simulink model "SistemaGrua021"  (R2020b)
settings: Solver=VariableStepAuto  StartTime=0.0  StopTime=10  RelTol=1e-3
values from neighbouring files (symbols this model uses):
  bcx = 1e6    (= 1000000)    [Valores_1.m]    (also in valoresPlanta.m; valoresPlanta_29_9_24.m; valoresPlanta_V3.m; valoresPlanta_v4.m)
  bcy = 1e7    (= 10000000)    [Valores_1.m]    (also in valoresPlanta.m; valoresPlanta_29_9_24.m; valoresPlanta_V3.m; valoresPlanta_v4.m)
  beq = bt+(btd+btm*it^2)/rtd^2    (= 21697.2)    [Valores.m]    (also in Valores_1.m; valoresPlanta_29_9_24.m; valoresPlanta_v4.m)
  bh_eq = bhm*ih^2+bhd    (= 8720)    [Valores.m]    (also in Valores_1.m; valoresPlanta.m; valoresPlanta_29_9_24.m; valoresPlanta_V3.m)
  bhb = 1e8    (= 100000000)    [Valores.m]    (also in Valores_1.m; valoresPlanta.m; valoresPlanta_29_9_24.m; valoresPlanta_V3.m)
  bhEb = 2.2e9    (= 2200000000)    [Valores.m]    (also in Valores_1.m; valoresPlanta.m; valoresPlanta_29_9_24.m; valoresPlanta_V3.m)
  btb = 5e6    (= 5000000)    [Valores.m]    (also in Valores_1.m; valoresPlanta.m; valoresPlanta_29_9_24.m; valoresPlanta_V3.m)
  bwu = 150    [Valores.m]    (also in Valores_1.m; valoresPlanta.m; valoresPlanta_29_9_24.m; valoresPlanta_V3.m)
  g = 9.80665    [Valores.m]    (also in Valores_1.m; valoresPlanta.m; valoresPlanta_29_9_24.m; valoresPlanta_V3.m)
  ih = 22    [Valores.m]    (also in Valores_1.m; valoresPlanta.m; valoresPlanta_29_9_24.m; valoresPlanta_V3.m)
  it = 30    [Valores.m]    (also in Valores_1.m; valoresPlanta.m; valoresPlanta_29_9_24.m; valoresPlanta_V3.m)
  Jh_eq = Jhm_hb*ih^2+Jhd_hEb    (= 18320)    [Valores.m]    (also in Valores_1.m; valoresPlanta.m; valoresPlanta_29_9_24.m; valoresPlanta_V3.m)
  kcy = 1.8e9    (= 1800000000)    [Valores_1.m]    (also in valoresPlanta.m; valoresPlanta_29_9_24.m; valoresPlanta_V3.m; valoresPlanta_v4.m)
  kwu = 2.36e8    (= 236000000)    [Valores.m]    (also in Valores_1.m; valoresPlanta.m; valoresPlanta_29_9_24.m; valoresPlanta_V3.m)
  Mc_max = 5e4    (= 50000)    [Valores.m]    (also in Valores_1.m; valoresPlanta.m; valoresPlanta_29_9_24.m; valoresPlanta_V3.m)
  Mc_min = 2e3    (= 2000)    [Valores.m]    (also in Valores_1.m; valoresPlanta.m; valoresPlanta_29_9_24.m; valoresPlanta_V3.m)
  Meq = Mt+(it^2*Jtm_tb+Jtd)/rtd^2    (= 60000)    [Valores.m]    (also in Valores_1.m; valoresPlanta_29_9_24.m; valoresPlanta_v4.m)
  rhd = 0.75    [Valores.m]    (also in Valores_1.m; valoresPlanta.m; valoresPlanta_29_9_24.m; valoresPlanta_V3.m)
  rtd = 0.5    [Valores.m]    (also in Valores_1.m; valoresPlanta.m; valoresPlanta_29_9_24.m; valoresPlanta_V3.m)
  tau_tm = 1e-3    (= 0.001)    [Valores.m]    (also in Valores_1.m; valoresPlanta.m; valoresPlanta_29_9_24.m; valoresPlanta_V3.m)
  tauhm = 1e-3    (= 0.001)    [Valores.m]    (also in Valores_1.m)
  Thb_Max = 5e4    (= 50000)    [Valores.m]    (also in Valores_1.m; valoresPlanta.m; valoresPlanta_29_9_24.m; valoresPlanta_V3.m)
  ThEb_Max = 1.1e6    (= 1100000)    [Valores.m]    (also in Valores_1.m; valoresPlanta.m; valoresPlanta_29_9_24.m; valoresPlanta_V3.m)
  Thm_Max = 2e4    (= 20000)    [Valores.m]    (also in Valores_1.m; valoresPlanta.m; valoresPlanta_29_9_24.m; valoresPlanta_V3.m)
  Ttb_Max = 5e3    (= 5000)    [Valores.m]    (also in Valores_1.m; valoresPlanta.m; valoresPlanta_29_9_24.m; valoresPlanta_V3.m)
  Ttm_Max = 3e3    (= 3000)    [Valores.m]    (also in Valores_1.m; valoresPlanta.m; valoresPlanta_29_9_24.m = 4000; valoresPlanta_V3.m)
  Yt0 = 45    [Valores.m]    (also in Valores_1.m; valoresPlanta.m; valoresPlanta_29_9_24.m; valoresPlanta_V3.m)
undefined symbols (not defined in the file or in its folder): sigbuilder_block
settings Model: Creator=Matias  LastModifiedBy=Matias

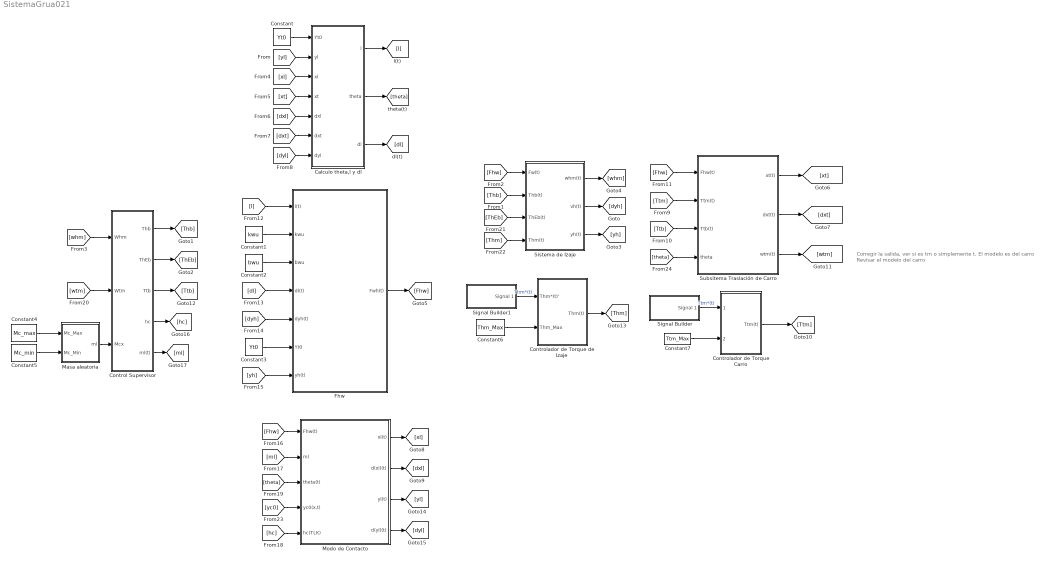
== system SistemaGrua021 ==
  note: Corregir la salida, ver si es tm o simplemente t. El modelo es del carro
      | Revisar el modelo del carro
  Calculo theta,l y dl : Subsystem
  Constant : Constant  Value=Yt0
  Constant1 : Constant  Value=kwu
  Constant2 : Constant  Value=bwu
  Constant3 : Constant  Value=Yt0
  Constant4 : Constant  Value=Mc_max
  Constant5 : Constant  Value=Mc_min
  Constant6 : Constant  Value=Thm_Max
  Constant7 : Constant  Value=Ttm_Max
  Control Supervisor : Subsystem
  Controlador de Torque Carro : Subsystem
  Controlador de Torque de Izaje : Subsystem
  Fhw : Subsystem
  Masa aleatoria : MATLAB Function  TreatAsAtomicUnit=on
  Modo de Contacto : Subsystem
  Signal Builder : Subsystem  Tag=STV Subsys  LoadFcn=sigbuilder_block('load');  StartFcn=sigbuilder_block('start');  StopFcn=sigbuilder_block('stop');  ClipboardFcn=sigbuilder_block('clipboard');  mask(Sigbuilder block){tuvar=[0:10]}
      mask help: Simulink:masks:SigbuilderBlock_MD
      mask init:
      | if ~strcmp(get_param(bdroot(gcbh),'SimulationStatus'),'stopped') tuvar = sigbuilder_block('maskInit'); end
      settings: CopyFcn=sigbuilder_block('copy');  DeleteFcn=sigbuilder_block('delete');  ModelCloseFcn=sigbuilder_block('modelClose');  PreSaveFcn=sigbuilder_block('preSave');  PauseFcn=sigbuilder_block('pause');  ContinueFcn=sigbuilder_block('continue');  NameChangeFcn=sigbuilder_block('namechange');  OpenFcn=sigbuilder_block('open',[5.4 36 1141.2 516.6 ]);  CloseFcn=sigbuilder_block('close');
      mask Display: plot(0, 0, 100, 100,[2, 2, 32, 32, 2], [68, 8, 8, 68, 68],[32, 2], [38, 38], [32, 19, 2],[53, 60, 44], [32, 17, 17, 2],[16, 16, 31, 31]);txt = getActiveGroup(gcbh);text(2, 100, txt,'verticalAlignment', 'top');
  Signal Builder1 : Subsystem  Tag=STV Subsys  LoadFcn=sigbuilder_block('load');  StartFcn=sigbuilder_block('start');  StopFcn=sigbuilder_block('stop');  ClipboardFcn=sigbuilder_block('clipboard');  mask(Sigbuilder block){tuvar=[0:10]}
      mask help: Simulink:masks:SigbuilderBlock_MD
      mask init:
      | if ~strcmp(get_param(bdroot(gcbh),'SimulationStatus'),'stopped') tuvar = sigbuilder_block('maskInit'); end
      settings: CopyFcn=sigbuilder_block('copy');  DeleteFcn=sigbuilder_block('delete');  ModelCloseFcn=sigbuilder_block('modelClose');  PreSaveFcn=sigbuilder_block('preSave');  PauseFcn=sigbuilder_block('pause');  ContinueFcn=sigbuilder_block('continue');  NameChangeFcn=sigbuilder_block('namechange');  OpenFcn=sigbuilder_block('open',[5.4 36 1141.2 516.6 ]);  CloseFcn=sigbuilder_block('close');
      mask Display: plot(0, 0, 100, 100,[2, 2, 32, 32, 2], [68, 8, 8, 68, 68],[32, 2], [38, 38], [32, 19, 2],[53, 60, 44], [32, 17, 17, 2],[16, 16, 31, 31]);txt = getActiveGroup(gcbh);text(2, 100, txt,'verticalAlignment', 'top');
  Sistema de Izaje : Subsystem
  Subsitema Traslación de Carro : Subsystem
  wires:
  [whm] -> Control Supervisor/1(Whm)
  Control Supervisor/1(Thb) -> [Thb]
  [Thb] -> Sistema de Izaje/2(Thb(t))
  [Fhw] -> Sistema de Izaje/1(Fw(t))
  Control Supervisor/2(ThEb) -> [ThEb]
  Calculo theta,l y dl/1(l) -> [l]
  Calculo theta,l y dl/2(theta) -> [theta]
  Constant/1 -> Calculo theta,l y dl/1(Yt0)
  [xt] -> Calculo theta,l y dl/4(xt)
  [xl] -> Calculo theta,l y dl/3(xl)
  [yl] -> Calculo theta,l y dl/2(yl)
  Calculo theta,l y dl/3(dl) -> [dl]
  [dyl] -> Calculo theta,l y dl/7(dyl)
  [dxt] -> Calculo theta,l y dl/6(dxt)
  [dxl] -> Calculo theta,l y dl/5(dxl)
  Fhw/1(Fwh(t)) -> [Fhw]
  [yh] -> Fhw/7(yh(t))
  [dyh] -> Fhw/5(dyh(t))
  [dl] -> Fhw/4(dl(t))
  [l] -> Fhw/1(l(t))
  Constant1/1 -> Fhw/2(kwu)
  Constant2/1 -> Fhw/3(bwu)
  [Ttb] -> Subsitema Traslación de Carro/3(Ttb(t))
  [Fhw] -> Subsitema Traslación de Carro/1(Fhw(t))
  [Ttm] -> Subsitema Traslación de Carro/2(Ttm(t))
  Subsitema Traslación de Carro/1(xt(t)) -> [xt]
  Subsitema Traslación de Carro/2(dxt(t)) -> [dxt]
  Controlador de Torque Carro/1(Ttm(t)) -> [Ttm]
  Signal Builder/1(Signal 1) -> Controlador de Torque Carro/1(Ttm*(t))  "Ttm*(t)"
  Subsitema Traslación de Carro/3(wtm(t)) -> [wtm]
  Control Supervisor/3(Ttb) -> [Ttb]
  [wtm] -> Control Supervisor/2(Wtm)
  Controlador de Torque de Izaje/1(Thm(t)) -> [Thm]
  Signal Builder1/1(Signal 1) -> Controlador de Torque de Izaje/1(Thm*(t)')  "Thm*(t)"
  Sistema de Izaje/1(whm(t)) -> [whm]
  Sistema de Izaje/2(vh(t)) -> [dyh]
  Sistema de Izaje/3(yh(t)) -> [yh]
  [ThEb] -> Sistema de Izaje/3(ThEb(t))
  [Thm] -> Sistema de Izaje/4(Thm(t))
  Constant3/1 -> Fhw/6(Yt0)
  Constant5/1 -> Masa aleatoria/2(Mc_Min)
  Constant4/1 -> Masa aleatoria/1(Mc_Max)
  Masa aleatoria/1(ml) -> Control Supervisor/3(Mcx)
  Constant6/1 -> Controlador de Torque de Izaje/2(Thm_Max)
  Constant7/1 -> Controlador de Torque Carro/2(Ttm_Max)
  [theta] -> Subsitema Traslación de Carro/4(theta)
  [yc0] -> Modo de Contacto/4(yc0(x,t))
  Modo de Contacto/2(d(xl)(t)) -> [dxl]
  Modo de Contacto/1(xl(t)) -> [xl]
  [hc] -> Modo de Contacto/5(hc(TLK))
  Modo de Contacto/4(d(yl)(t)) -> [dyl]
  [theta] -> Modo de Contacto/3(theta(t))
  Modo de Contacto/3(yl(t)) -> [yl]
  [ml] -> Modo de Contacto/2(ml)
  [Fhw] -> Modo de Contacto/1(Fhw(t))
  Control Supervisor/5(ml(t)) -> [ml]
  Control Supervisor/4(hc) -> [hc]

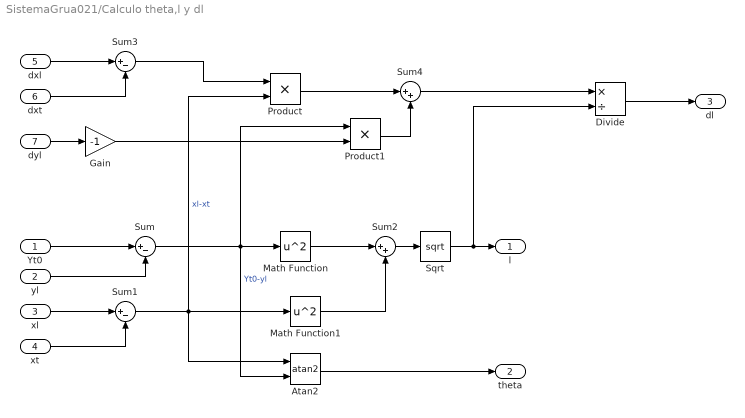
== system SistemaGrua021/Calculo theta,l y dl ==
  Yt0 : Inport
  yl : Inport  Port=2
  xl : Inport  Port=3
  xt : Inport  Port=4
  dxl : Inport  Port=5
  dxt : Inport  Port=6
  dyl : Inport  Port=7
  Atan2 : Trigonometry  Operator=atan2
  Divide : Product  Inputs=*/
  Gain : Gain  Gain=-1
  Math Function : Math  Operator=square  SaturateOnIntegerOverflow=on
  Math Function1 : Math  Operator=square  SaturateOnIntegerOverflow=on
  Product : Product
  Product1 : Product
  Sqrt : Sqrt  SaturateOnIntegerOverflow=on
  Sum : Sum  Inputs=|+-
  Sum1 : Sum  Inputs=|+-
  Sum2 : Sum  Inputs=|++
  Sum3 : Sum  Inputs=|+-
  Sum4 : Sum  Inputs=|++
  l : Outport
  theta : Outport  Port=2
  dl : Outport  Port=3
  wires:
  Yt0/1 -> Sum/1
  yl/1 -> Sum/2
  xl/1 -> Sum1/1
  xt/1 -> Sum1/2
  Atan2/1 -> theta/1
  Sum1/1 -> Product/2, Math Function1/1, Atan2/1  "xl-xt"
  Sum/1 -> Product1/1, Atan2/2, Math Function/1  "Yt0-yl"
  Math Function/1 -> Sum2/1
  Math Function1/1 -> Sum2/2
  Sum2/1 -> Sqrt/1
  Sqrt/1 -> Divide/2, l/1
  dxl/1 -> Sum3/1
  dxt/1 -> Sum3/2
  Sum3/1 -> Product/1
  dyl/1 -> Gain/1
  Gain/1 -> Product1/2
  Product/1 -> Sum4/1
  Product1/1 -> Sum4/2
  Sum4/1 -> Divide/1
  Divide/1 -> dl/1

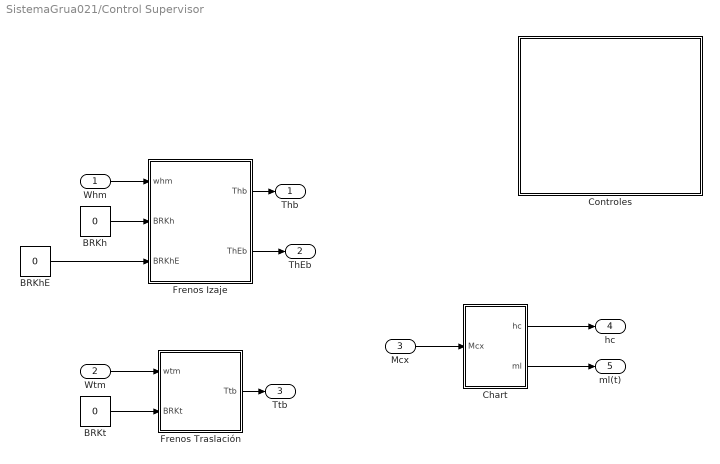
== system SistemaGrua021/Control Supervisor ==
  Whm : Inport
  Wtm : Inport  Port=2
  Mcx : Inport  Port=3
  BRKh : Constant  Value=0
  BRKhE : Constant  Value=0
  BRKt : Constant  Value=0
  Chart : Stateflow chart  TreatAsAtomicUnit=on
  Controles : Subsystem
  "Frenos Izaje " : Stateflow chart  TreatAsAtomicUnit=on
  Frenos Traslación : Stateflow chart  TreatAsAtomicUnit=on
  Thb : Outport
  ThEb : Outport  Port=2
  Ttb : Outport  Port=3
  hc : Outport  Port=4
  ml(t) : Outport  Port=5
  wires:
  "Frenos Izaje "/1(Thb) -> Thb/1
  BRKh/1 -> "Frenos Izaje "/2(BRKh)
  Whm/1 -> "Frenos Izaje "/1(whm)
  BRKhE/1 -> "Frenos Izaje "/3(BRKhE)
  "Frenos Izaje "/2(ThEb) -> ThEb/1
  Wtm/1 -> Frenos Traslación/1(wtm)
  Frenos Traslación/1(Ttb) -> Ttb/1
  BRKt/1 -> Frenos Traslación/2(BRKt)
  Chart/2(ml) -> ml(t)/1
  Chart/1(hc) -> hc/1
  Mcx/1 -> Chart/1(Mcx)

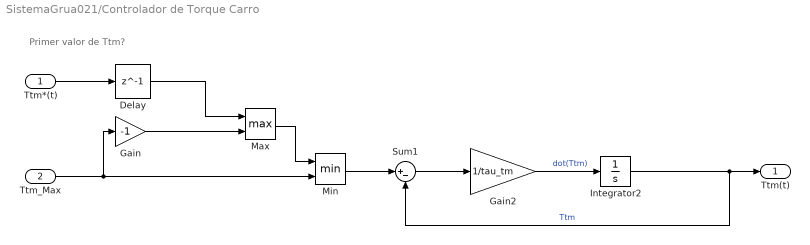
== system SistemaGrua021/Controlador de Torque Carro ==
  note: Primer valor de Ttm?
  Ttm*(t) : Inport
  Ttm_Max : Inport  Port=2
  Delay : Delay  DelayLength=1  InitialCondition=0
  Gain : Gain  Gain=-1
  Gain2 : Gain  Gain=1/tau_tm
  Integrator2 : Integrator
  Max : MinMax  Function=max  Inputs=2
  Min : MinMax  Inputs=2
  Sum1 : Sum  Inputs=|+-
  Ttm(t) : Outport
  wires:
  Integrator2/1 -> Ttm(t)/1, Sum1/2  "Ttm"
  Sum1/1 -> Gain2/1
  Gain2/1 -> Integrator2/1  "dot(Ttm)"
  Ttm*(t)/1 -> Delay/1
  Gain/1 -> Max/2
  Delay/1 -> Max/1
  Max/1 -> Min/1
  Min/1 -> Sum1/1
  Ttm_Max/1 -> Gain/1, Min/2

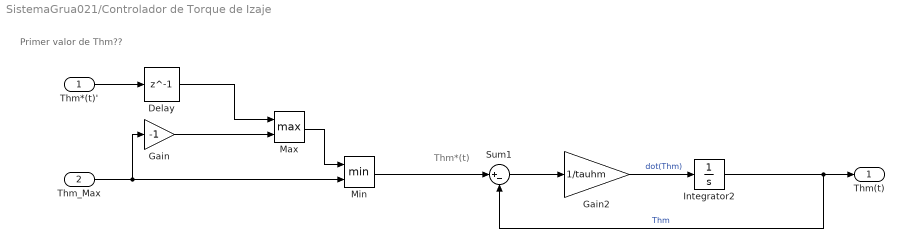
== system SistemaGrua021/Controlador de Torque de Izaje ==
  note: Primer valor de Thm??
  note: Thm*(t)
  Thm*(t)' : Inport
  Thm_Max : Inport  Port=2
  Delay : Delay  DelayLength=1  InitialCondition=0
  Gain : Gain  Gain=-1
  Gain2 : Gain  Gain=1/tauhm
  Integrator2 : Integrator
  Max : MinMax  Function=max  Inputs=2
  Min : MinMax  Inputs=2
  Sum1 : Sum  Inputs=|+-
  Thm(t) : Outport
  wires:
  Integrator2/1 -> Thm(t)/1, Sum1/2  "Thm"
  Thm*(t)'/1 -> Delay/1
  Sum1/1 -> Gain2/1
  Gain2/1 -> Integrator2/1  "dot(Thm)"
  Thm_Max/1 -> Gain/1, Min/2
  Gain/1 -> Max/2
  Delay/1 -> Max/1
  Max/1 -> Min/1
  Min/1 -> Sum1/1

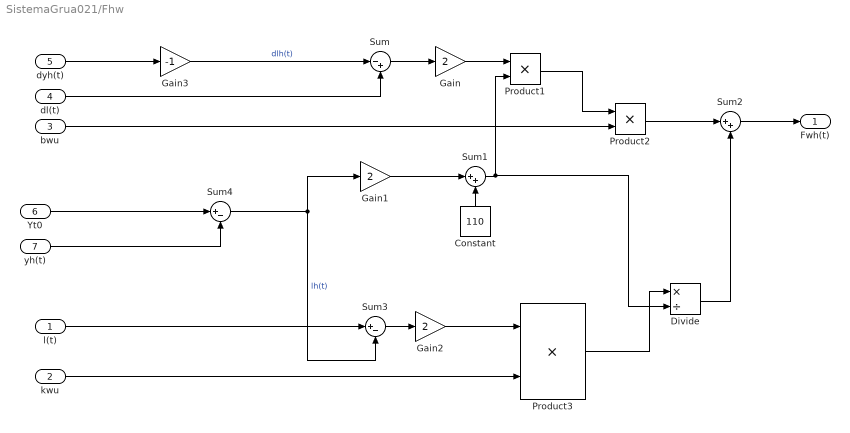
== system SistemaGrua021/Fhw ==
  l(t) : Inport
  kwu : Inport  Port=2
  bwu : Inport  Port=3
  dl(t) : Inport  Port=4
  dyh(t) : Inport  Port=5
  Yt0 : Inport  Port=6
  yh(t) : Inport  Port=7
  Constant : Constant  Value=110
  Divide : Product  Inputs=*/
  Gain : Gain  Gain=2
  Gain1 : Gain  Gain=2
  Gain2 : Gain  Gain=2
  Gain3 : Gain  Gain=-1
  Product1 : Product
  Product2 : Product
  Product3 : Product
  Sum : Sum  Inputs=|-+
  Sum1 : Sum  Inputs=|++
  Sum2 : Sum  Inputs=|++
  Sum3 : Sum  Inputs=|+-
  Sum4 : Sum  Inputs=|+-
  Fwh(t) : Outport
  wires:
  dl(t)/1 -> Sum/2
  Sum/1 -> Gain/1
  Gain1/1 -> Sum1/1
  Sum4/1 -> Sum3/2, Gain1/1  "lh(t)"
  l(t)/1 -> Sum3/1
  Constant/1 -> Sum1/2
  Gain/1 -> Product1/1
  Sum1/1 -> Product1/2, Divide/2
  Product1/1 -> Product2/1
  bwu/1 -> Product2/2
  Product2/1 -> Sum2/1
  Sum3/1 -> Gain2/1
  Gain2/1 -> Product3/1
  kwu/1 -> Product3/2
  Product3/1 -> Divide/1
  Divide/1 -> Sum2/2
  Sum2/1 -> Fwh(t)/1
  dyh(t)/1 -> Gain3/1
  Gain3/1 -> Sum/1  "dlh(t)"
  Yt0/1 -> Sum4/1
  yh(t)/1 -> Sum4/2

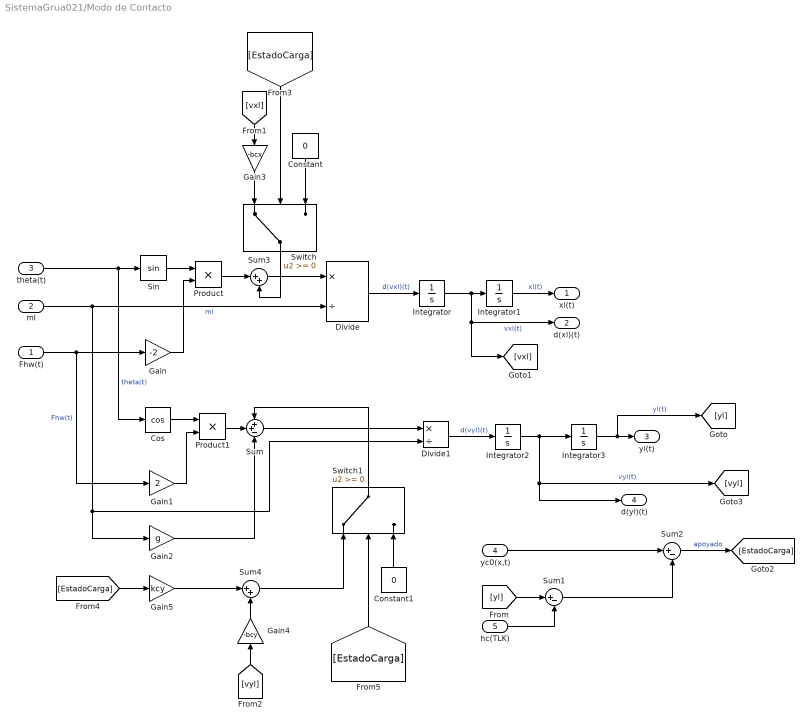
== system SistemaGrua021/Modo de Contacto ==
  Fhw(t) : Inport
  ml : Inport  Port=2
  theta(t) : Inport  Port=3
  yc0(x,t) : Inport  Port=4
  hc(TLK) : Inport  Port=5
  Constant : Constant  Value=0
  Constant1 : Constant  Value=0
  Cos : Trigonometry  Operator=cos
  Divide : Product  Inputs=*/
  Divide1 : Product  Inputs=*/
  Gain : Gain  Gain=-2
  Gain1 : Gain  Gain=2
  Gain2 : Gain  Gain=g
  Gain3 : Gain  Gain=-bcx
  Gain4 : Gain  Gain=-bcy
  Gain5 : Gain  Gain=kcy
  Integrator{,1..3} (4 alike) : Integrator
  Product : Product
  Product1 : Product
  Sin : Trigonometry
  Sum : Sum  Inputs=++-
  Sum1 : Sum  Inputs=|+-
  Sum2 : Sum  Inputs=|+-
  Sum3 : Sum  Inputs=|++
  Sum4 : Sum  Inputs=|++
  Switch : Switch
  Switch1 : Switch
  xl(t) : Outport
  d(xl)(t) : Outport  Port=2
  yl(t) : Outport  Port=3
  d(yl)(t) : Outport  Port=4
  wires:
  theta(t)/1 -> Sin/1, Cos/1  "theta(t)"
  Fhw(t)/1 -> Gain/1, Gain1/1  "Fhw(t)"
  Sin/1 -> Product/1
  Gain/1 -> Product/2
  ml/1 -> Gain2/1, Divide1/2, Divide/2  "ml"
  Divide/1 -> Integrator/1  "d(vxl)(t)"
  Integrator1/1 -> xl(t)/1  "xl(t)"
  Cos/1 -> Product1/1
  Gain1/1 -> Product1/2
  Divide1/1 -> Integrator2/1  "d(vyl)(t)"
  Integrator3/1 -> [yl], yl(t)/1  "yl(t)"
  Integrator/1 -> Integrator1/1, [vxl], d(xl)(t)/1  "vxl(t)"
  Integrator2/1 -> Integrator3/1, [vyl], d(yl)(t)/1  "vyl(t)"
  hc(TLK)/1 -> Sum1/2
  [yl] -> Sum1/1
  yc0(x,t)/1 -> Sum2/1
  Sum1/1 -> Sum2/2
  Product/1 -> Sum3/1
  Sum3/1 -> Divide/1
  Switch/1 -> Sum3/2
  [vxl] -> Gain3/1
  Sum/1 -> Divide1/1
  Product1/1 -> Sum/2
  Gain2/1 -> Sum/3
  [vyl] -> Gain4/1
  Switch1/1 -> Sum/1
  Sum2/1 -> [EstadoCarga]  "apoyado"
  [EstadoCarga] -> Switch/2
  Gain4/1 -> Sum4/2
  [EstadoCarga] -> Gain5/1
  Gain5/1 -> Sum4/1
  [EstadoCarga] -> Switch1/2
  Constant/1 -> Switch/3
  Gain3/1 -> Switch/1
  Constant1/1 -> Switch1/3
  Sum4/1 -> Switch1/1

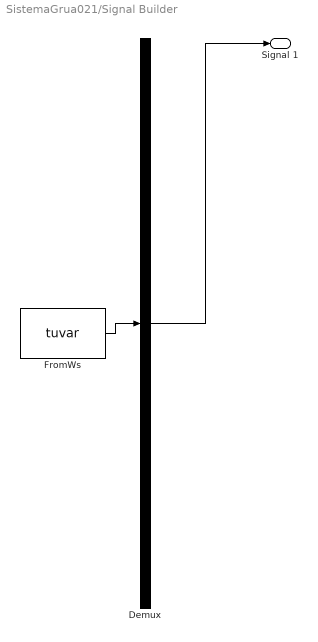
== system SistemaGrua021/Signal Builder ==
  Demux : Demux  Tag=STV Demux  Outputs=1
      settings: DisplayOption=none
  FromWs : FromWorkspace  Tag=STV FromWs  VariableName=tuvar
      SigBuilderData=|
      | common.afterFinalStr = 'Extrapolate'
      | common.sampleTime = 0
      | dataSet.timeRange = [0 10]
      | dataSet.name = 'Group 1'
      | sbobj.Groups.Name = 'Group 1'
      | sbobj.Groups.Signals.Name = 'Signal 1'
      | sbobj.Groups.Signals.XData = [0 4 6 10]
      | sbobj.Groups.Signals.YData = [0 20000 20000 0]
  Signal 1 : Outport  Tag=STV Outport
  wires:
  Demux/1 -> Signal 1/1
  FromWs/1 -> Demux/1

== system SistemaGrua021/Signal Builder1 ==
  Demux : Demux  Tag=STV Demux  Outputs=1
      settings: DisplayOption=none
  FromWs : FromWorkspace  Tag=STV FromWs  VariableName=tuvar
      SigBuilderData=|
      | common.afterFinalStr = 'Extrapolate'
      | common.sampleTime = 0
      | dataSet.timeRange = [0 10]
      | dataSet.name = 'Group 1'
      | sbobj.Groups.Name = 'Group 1'
      | sbobj.Groups.Signals.Name = 'Signal 1'
      | sbobj.Groups.Signals.XData = [0 4 6 10]
      | sbobj.Groups.Signals.YData = [0 20000 20000 0]
  Signal 1 : Outport  Tag=STV Outport
  wires:
  Demux/1 -> Signal 1/1
  FromWs/1 -> Demux/1

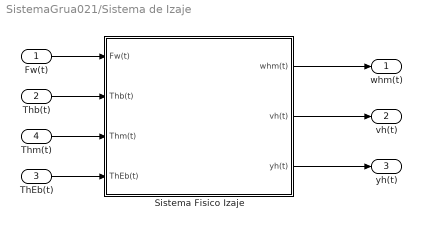
== system SistemaGrua021/Sistema de Izaje ==
  Fw(t) : Inport
  Thb(t) : Inport  Port=2
  ThEb(t) : Inport  Port=3
  Thm(t) : Inport  Port=4
  Sistema Fisico Izaje : Subsystem
  whm(t) : Outport
  vh(t) : Outport  Port=2
  yh(t) : Outport  Port=3
  wires:
  Fw(t)/1 -> Sistema Fisico Izaje/1(Fw(t))
  Thb(t)/1 -> Sistema Fisico Izaje/2(Thb(t))
  Thm(t)/1 -> Sistema Fisico Izaje/3(Thm(t))
  Sistema Fisico Izaje/1(whm(t)) -> whm(t)/1
  Sistema Fisico Izaje/2(vh(t)) -> vh(t)/1
  Sistema Fisico Izaje/3(yh(t)) -> yh(t)/1
  ThEb(t)/1 -> Sistema Fisico Izaje/4(ThEb(t))

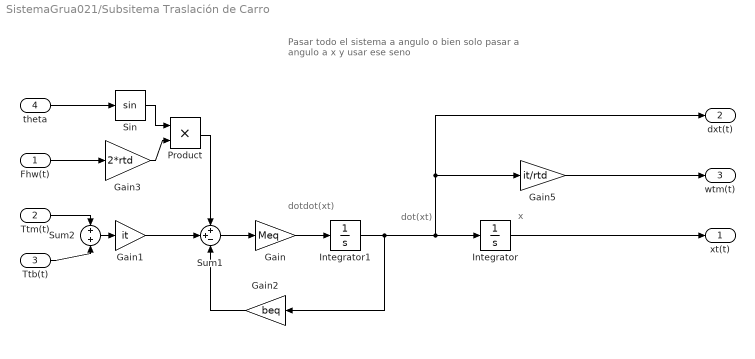
== system SistemaGrua021/Subsitema Traslación de Carro ==
  note: x
  note: dot(xt)
  note: dotdot(xt)
  note: Pasar todo el sistema a angulo
      | o bien solo pasar a angulo a x y usar ese seno
  Fhw(t) : Inport
  Ttm(t) : Inport  Port=2
  Ttb(t) : Inport  Port=3
  theta : Inport  Port=4
  Gain : Gain  Gain=Meq
  Gain1 : Gain  Gain=it
  Gain2 : Gain  Gain=beq
  Gain3 : Gain  Gain=2*rtd
  Gain5 : Gain  Gain=it/rtd
  Integrator : Integrator
  Integrator1 : Integrator
  Product : Product
  Sin : Trigonometry
  Sum1 : Sum  Inputs=++-
  Sum2 : Sum
  xt(t) : Outport
  dxt(t) : Outport  Port=2
  wtm(t) : Outport  Port=3
  wires:
  Sin/1 -> Product/1
  Gain1/1 -> Sum1/2
  Integrator1/1 -> Gain2/1, dxt(t)/1, Gain5/1, Integrator/1
  Sum2/1 -> Gain1/1
  Gain3/1 -> Product/2
  Gain2/1 -> Sum1/3
  Gain/1 -> Integrator1/1
  Sum1/1 -> Gain/1
  Product/1 -> Sum1/1
  Fhw(t)/1 -> Gain3/1
  Ttb(t)/1 -> Sum2/2
  Ttm(t)/1 -> Sum2/1
  Gain5/1 -> wtm(t)/1
  Integrator/1 -> xt(t)/1
  theta/1 -> Sin/1

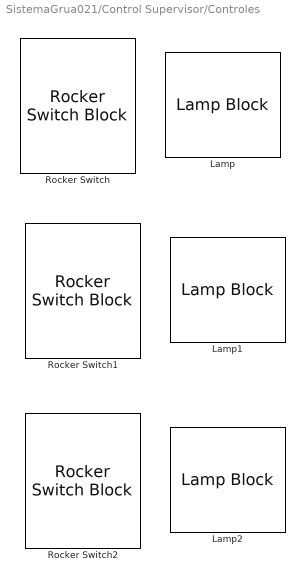
== system SistemaGrua021/Control Supervisor/Controles ==
  Lamp : LampBlock
  Lamp1 : LampBlock
  Lamp2 : LampBlock
  Rocker Switch : RockerSwitchBlock
      settings: Values={{'Off', 'On'}, [0 1]}
  Rocker Switch1 : RockerSwitchBlock
      settings: Values={{'Off', 'On'}, [0 1]}
  Rocker Switch2 : RockerSwitchBlock
      settings: Values={{'Off', 'On'}, [0 1]}

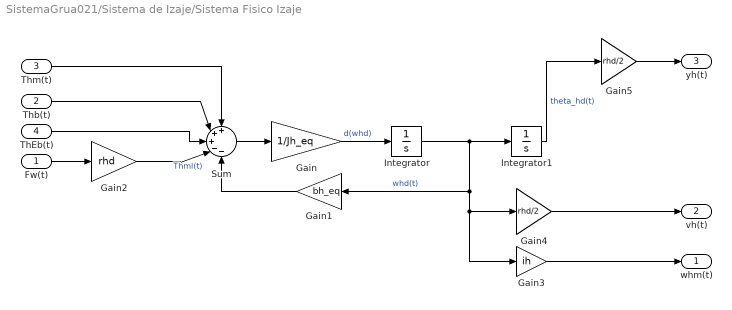
== system SistemaGrua021/Sistema de Izaje/Sistema Fisico Izaje ==
  Fw(t) : Inport
  Thb(t) : Inport  Port=2
  Thm(t) : Inport  Port=3
  ThEb(t) : Inport  Port=4
  Gain : Gain  Gain=1/Jh_eq
  Gain1 : Gain  Gain=bh_eq
  Gain2 : Gain  Gain=rhd
  Gain3 : Gain  Gain=ih
  Gain4 : Gain  Gain=rhd/2
  Gain5 : Gain  Gain=rhd/2
  Integrator : Integrator
  Integrator1 : Integrator
  Sum : Sum  Inputs=+++--
  whm(t) : Outport
  vh(t) : Outport  Port=2
  yh(t) : Outport  Port=3
  wires:
  Gain/1 -> Integrator/1  "d(whd)"
  Sum/1 -> Gain/1
  Integrator/1 -> Gain3/1, Gain4/1, Gain1/1, Integrator1/1  "whd(t)"
  Fw(t)/1 -> Gain2/1
  Thb(t)/1 -> Sum/2
  Thm(t)/1 -> Sum/1
  Gain1/1 -> Sum/5
  Gain2/1 -> Sum/4  "Thml(t)"
  ThEb(t)/1 -> Sum/3
  Gain3/1 -> whm(t)/1
  Gain4/1 -> vh(t)/1
  Integrator1/1 -> Gain5/1  "theta_hd(t)"
  Gain5/1 -> yh(t)/1

== stateflow chart SistemaGrua021/Control Supervisor/Frenos Traslación ==
  state FrenosOperacion
    state BRKt_off
      during:
      Ttb=-btb*wtm;
      Ttb=min(Ttb_Max,Ttb);
    state BRKt_on
      during:
      Ttb=0;
    (default) -> BRKt_off
    BRKt_off -> BRKt_on : [BRKt==1 ]
    BRKt_on -> BRKt_off : [BRKt==0]
  data: Ttb output; wtm input; btb parameter; Ttb_Max parameter; BRKt input

== stateflow chart SistemaGrua021/Control Supervisor/Chart ==
  state TLK_OFF
    during:
    hc=0;
    ml=Ms;
  state TLK_ON
    during:
    hc=2.5;
    ml=Ms+Mcx;
  (default) -> TLK_OFF
  TLK_OFF -> TLK_ON : [Mcx>0]
  TLK_ON -> TLK_OFF : [Mcx<=0]
  data: Mcx input; hc output; ml output; Ms parameter

== stateflow chart SistemaGrua021/Control Supervisor/Frenos Izaje  ==
  state FrenosOperacion
    state BRKh_off
      during:
      Thb=-bhb*whm;
      Thb=min(Thb_Max,Thb);
    state BRKh_on
      during:
      Thb=0;
    (default) -> BRKh_off
    BRKh_off -> BRKh_on [order 1] : [BRKh==1 && BRKhE==1]
    BRKh_on -> BRKh_off [order 1] : [BRKh==0 && BRKhE==1]
  state FrenosEmergencia
    state BRKhE_off
      during:
      ThEb=-bhEb*whm;
      ThEb=min(ThEb_Max,ThEb);
    state BRKhE_on
      during:
      ThEb=0;
    (default) -> BRKhE_off
    BRKhE_off -> BRKhE_on : [BRKhE==1]
    BRKhE_on -> BRKhE_off [order 1] : [BRKhE==0]
  BRKh_on -> FrenosEmergencia [order 2] : [BRKhE==0]
  BRKh_off -> FrenosEmergencia [order 2] : [BRKhE==0]
  BRKhE_on -> FrenosOperacion [order 2] : [BRKhE==1]
  (default) -> FrenosEmergencia
  data: Thb output; whm input; bhb parameter; Thb_Max parameter; BRKh input; ThEb output; bhEb parameter; ThEb_Max parameter; BRKhE input

== matlab function SistemaGrua021/Masa aleatoria ==
  data: Mc_Max input; ml output; Mc_Min input
function ml = fcn(Mc_Max, Mc_Min)
%Cambiar los valores de tiempo a criterio
tic;
while (1)
    tic;
    t = randi([5,8],1);
    elapsed_time = toc;
    %elapsed_time = end_time - start_time;
    while elapsed_time < t
        ml = Mc_Min + (Mc_Max - Mc_Min)*rand(1); %genero numero aleatorio
        %disp(ml);
        pause(1);
        elapsed_time = elapsed_time + toc;
    end
    %fprintf("Masa excedida")
    ml = Mc_Max + 0.01 * randi([1,15],1) * Mc_Max;   %genero aleatorio con sobrecarga (hasta 15% mas)
    %disp(ml);
    pause(1);   %Pausa de 5 segundos
    elapsed_time = 0;
end
